simulink library "lib_Convection_MixedConv"  (R2015a)
settings: Solver=ode45  StartTime=0.0  StopTime=10.0  RelTol=1e-3
settings Model: Creator=jlkratz  LastModifiedBy=jlkratz

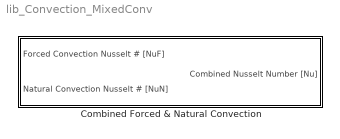
== system lib_Convection_MixedConv ==
  Combined Forced & Natural Convection : Subsystem  mask(TSAT: Combined Forced & Natural Convection Block){dir_M=on, n_M=3}
      mask prompts: dir_M "dir_M - Flow direction (checked - assisted or transverse flow, unchecked - opposing flow)"; n_M "n_M - Correlation exponent"
      mask help: This block can be used to approximate the combined forced and natural convection Nusselt number. This block is most useful for scenarios where neither forced or natural convection is negligible. Three special cases have been extensively studied corresonding to assisted flow (buoyancy force is acting in the same direction as the forced flow), transverse flow (buoyancy force is acting in a direction perpendicular to the forced flow), and opposing flow (buoyancy forced are acting in the opposite direction of the forced flow). In the cases of assisting flow and transfer flow the buoyancy forces are enhancing the rate of heat transfer while opposing flow will decrease it. For more information on the equation used to approximate the mixed Nusselt number, refer to the block help menu.
      mask Help: web(which('Convection_TSAT_MixedConv.html'),'-helpbrowser')

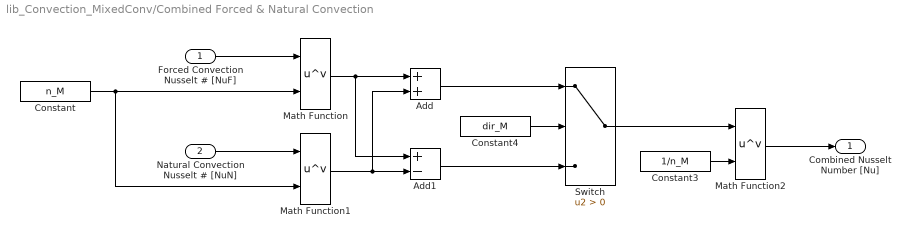
== system lib_Convection_MixedConv/Combined Forced & Natural Convection ==
  "Forced Convection Nusselt # [NuF] " : Inport
  Natural Convection Nusselt # [NuN] : Inport  Port=2
  Add : Sum
  Add1 : Sum  Inputs=+-
  Constant : Constant  Value=n_M
  Constant3 : Constant  Value=1/n_M
  Constant4 : Constant  Value=dir_M
  Math Function : Math  Operator=pow  SaturateOnIntegerOverflow=on
  Math Function1 : Math  Operator=pow  SaturateOnIntegerOverflow=on
  Math Function2 : Math  Operator=pow  SaturateOnIntegerOverflow=on
  Switch : Switch  Criteria=u2 > Threshold
  Combined Nusselt Number [Nu] : Outport
  wires:
  Natural Convection Nusselt # [NuN]/1 -> Math Function1/1
  Constant3/1 -> Math Function2/2
  Constant4/1 -> Switch/2
  Add/1 -> Switch/1
  Switch/1 -> Math Function2/1
  Constant/1 -> Math Function1/2, Math Function/2
  Add1/1 -> Switch/3
  Math Function1/1 -> Add1/2, Add/2
  "Forced Convection Nusselt # [NuF] "/1 -> Math Function/1
  Math Function/1 -> Add/1, Add1/1
  Math Function2/1 -> Combined Nusselt Number [Nu]/1
